simulink model "MagicFormulaTyreLibrary_SimulinkExample"  (R2021a)
settings: Solver=FixedStepDiscrete  StartTime=0.0  StopTime=2  FixedStep=0.01  RelTol=1e-3
libraries: MagicFormulaTyreLibrary x1, simulink x1
settings Model: Creator=Tom  LastModifiedBy=Tom

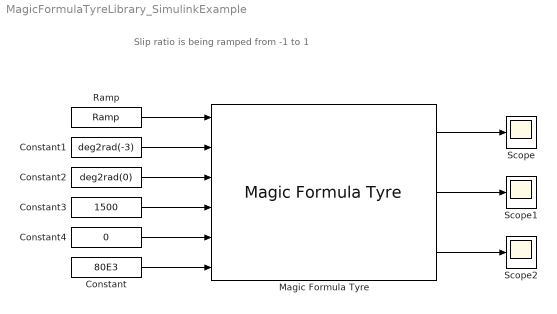
== system MagicFormulaTyreLibrary_SimulinkExample ==
  note: Slip ratio is being ramped from -1 to 1
  Constant : Constant  Value=80E3
  Constant1 : Constant  Value=deg2rad(-3)
  Constant2 : Constant  Value=deg2rad(0)
  Constant3 : Constant  Value=1500
  Constant4 : Constant  Value=0
  Magic Formula Tyre : MagicFormulaTyreLibrary/Magic Formula Tyre  file='doc/examples/fsae-ttc-data/fsaettc_obfuscated.tir'  p=struct()  usemode=0
  Ramp : simulink/Sources/Ramp  slope=1  start=0  InitialOutput=-1
  Scope : Scope
  Scope1 : Scope
  Scope2 : Scope
  wires:
  Magic Formula Tyre/2 -> Scope1/1
  Magic Formula Tyre/3 -> Scope2/1
  Ramp/1 -> Magic Formula Tyre/1
  Constant/1 -> Magic Formula Tyre/6
  Constant1/1 -> Magic Formula Tyre/2
  Constant2/1 -> Magic Formula Tyre/3
  Constant3/1 -> Magic Formula Tyre/4
  Constant4/1 -> Magic Formula Tyre/5
  Magic Formula Tyre/1 -> Scope/1
